simulink model "module_8_exercise_2"  (R2022a)
settings: Solver=FixedStepAuto  StartTime=0.0  StopTime=30  FixedStep=0.01  RelTol=1e-3
libraries: simulink x1
settings Model: Creator=hntran  LastModifiedBy=hntran

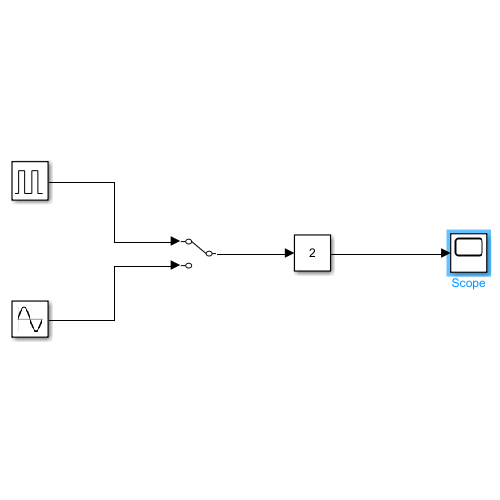
[thumbnail: Simulink's stored preview of the top-level diagram]
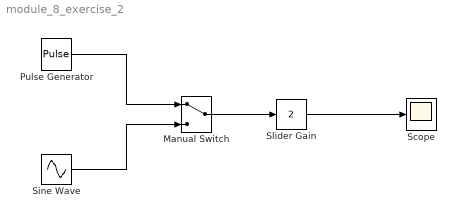
== system module_8_exercise_2 ==
  Manual Switch : ManualSwitch
  Pulse Generator : DiscretePulseGenerator  PulseType=Time based  Period=10  PulseWidth=40
  Scope : Scope
  Sine Wave : Sin  Amplitude=2  Frequency=2  SampleTime=0
  Slider Gain : simulink/Math Operations/Slider Gain  gain=2  low=-10  high=10
  wires:
  Slider Gain/1 -> Scope/1
  Manual Switch/1 -> Slider Gain/1
  Pulse Generator/1 -> Manual Switch/1
  Sine Wave/1 -> Manual Switch/2
